simulink model "newsyscase1modctrlflowmod"  (R2014b)
settings: Solver=ode45  StartTime=0.0  StopTime=2000  RelTol=1e-3
values from neighbouring files (symbols this model uses):
  Dsteptime = 1000    [mainrun.m]
undefined symbols (not defined in the file or in its folder): D1, D10, D11, D12, D2, D3, D4, D5, D6, D7, D8, D9, Is1, Is2, Is3, Is4, Ks1, Ks2, Ks3, Ks4
undefined symbols (not defined in the file): H1C1initT, H1C2initT, H2C1initT, H2C2initT, H2C3initT, Ttank1, Ttank2, Ttank3, Ttank4, Ttank5
libraries: simulink x4, commblkintrlv2 x1
settings Model: Creator=fredrik  LastModifiedBy=fredrik

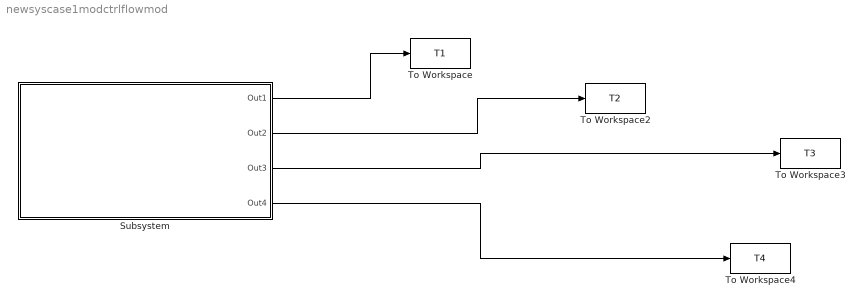
== system newsyscase1modctrlflowmod ==
  Subsystem : Subsystem
  To Workspace : ToWorkspace  VariableName=T1  SaveFormat=Timeseries  SampleTime=-1
  To Workspace2 : ToWorkspace  VariableName=T2  SaveFormat=Timeseries  SampleTime=-1
  To Workspace3 : ToWorkspace  VariableName=T3  SaveFormat=Timeseries  SampleTime=-1
  To Workspace4 : ToWorkspace  VariableName=T4  SaveFormat=Timeseries  SampleTime=-1
  wires:
  Subsystem/1(Out1) -> To Workspace/1
  Subsystem/2(Out2) -> To Workspace2/1
  Subsystem/3(Out3) -> To Workspace3/1
  Subsystem/4(Out4) -> To Workspace4/1

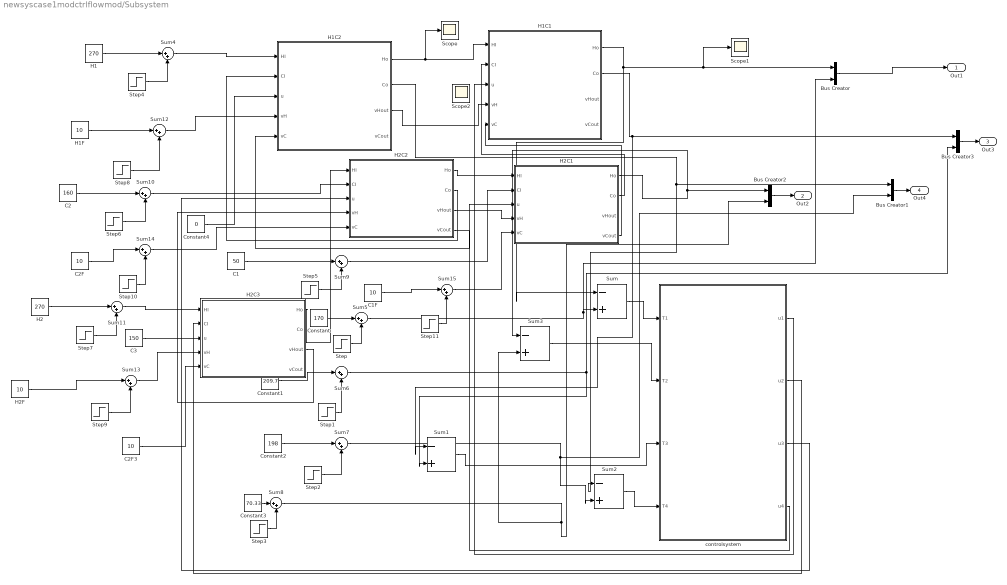
== system newsyscase1modctrlflowmod/Subsystem ==
  Bus Creator{,1..3} (4 alike) : BusCreator  Inputs=2
  C1 : Constant  Value=50
  C1F : Constant  Value=10
  C2 : Constant  Value=160
  C2F : Constant  Value=10
  C2F3 : Constant  Value=10
  C3 : Constant  Value=150
  Constant : Constant  Value=170
  Constant1 : Constant  Value=209.7
  Constant2 : Constant  Value=198
  Constant3 : Constant  Value=70.33
  Constant4 : Constant  Value=0
  H1 : Constant  Value=270
  H1C1 : Subsystem  mask{A=239.1281493, Vhot=Ttank2*10, Vcold=Ttank2*10, Q=1000, Ulm=0.5, Thin=225.55555, Thout=170, Tcin=160, Tcout=210, vh=10, vc=10, n=10, initT=H1C1initT, hot=1}
      mask prompts: A "Area"; Vhot "Volume for hot stream"; Vcold "Volume for cold stream"; Ulm "U"; Thin "Hotin"; Thout "Hotout"; Tcin "Coldin"; Tcout "Coldout"; vh "Rated hot flow"; vc "Rated cold flow"; n "Number of cells"; initT "initial temperature"; hot "1 if hot bypass, 0 if cold"
      mask init:
      | % vH=sym('vH');
      | % Vh=sym('Vh');
      | % th=sym('th');
      | % u0=sym('u0'); %
      | % Vend=sym('Vend');
      | % vC=sym('vC');
      | % Vc=sym('Vc');
      | % tc=sym('tc');
      | 
      | %%tank1:
      | 
      | %% E-2401
      | Fc=Q/(Tcout-Tcin)/vc;
      | Fh=Q/(Thin-Thout)/vh;
      | %Fsak=2*1/(1/Fc+1/Fh);
      | %Nth=Ulm*A/Fsak;
      | %U=Ulm/(n-Nth)*n;
      | %UA=A*U;
      | tc=1/(A/(Fc*Vcold));%cold constant for transfer
      | th=1/(A/(Fh*Vhot));%hot constant for transfer
      | Am=zeros(2*n+1);
      | AU=zeros(2*n+1);
      | Avhot=zeros(2*n+1);
      | Avcold=zeros(2*n+1);
      | Ath=zeros(2*n+1);
      | B=zeros(2*n,1);
      | C=zeros(2,2*n+1);
      | if hot
      |     C(2,end)=1;
      |     C(1,2)=1;
      | else
      |     C(1,end)=1;
      |     C(2,end-2)=1;
      | end
      | D=zeros(2*n,1);
      | 
      | 
      | for k=1:2*n
      |     if mod(k,2) == 1
      |         Ath(k,k)=-1/th;
      |         Am(k,k)=-n/Vhot;
      |         Avhot(k,k)=1;
      |         Ath(k,k+1)=1/th;
      |         if hot
      |             AU(k,k)=n/Vhot;
      |         end
      |         if k~=1
      |             Am(k,k-2)=n/Vhot;
      |             if hot
      |                 AU(k,k-2)=-n/Vhot;
      |             end
      |         end
      |     else
      |         Ath(k,k)=-1/tc;
      |         Avcold(k,k)=1;
      |         Am(k,k)=-n/Vcold;
      |         Ath(k,k-1)=1/tc;
      |         if ~hot
      |             AU(k,k)=n/Vcold;
      |         end
      |         if k~=2*n
      |             Am(k,k+2)=n/Vcold;
      |             if ~hot
      |                 AU(k,k+2)=-n/Vcold;
      |             end
      |         end
      |     end
      | end
      | ADscold=zeros(2*n+1);
      | ADshot=zeros(2*n+1);
      | Ds=zeros(2*n+1,2);
      | %Ds=sym(Ds);
      | Ds(1,1)=(n/Vhot);
      | ADshot(1,1)=1;
      | Ds(2*n,2)=(n/Vcold);
      | ADscold(2*n,2*n)=1;
      | DsU=zeros(2*n+1,2);
      | %DsU=sym(DsU);
      | if hot
      |     DsU(1,1)=(-n/Vhot);
      | else
      |     DsU(2*n,2)=(-n/Vcold);
      | end
      | 
      | 
      | if hot
      |     Am(2*n+1,end-2)=n/Vhot;
      |     AU(2*n+1,end-2)=-n/Vhot;
      |     Am(2*n+1,end)=-n/Vhot;
      |     Avhot(end,end)=1;
      |     DsU(end,1)=n/Vhot;
      |     ADshot(end,end)=1;
      | else
      |     Am(2*n+1,2)=n/Vcold;
      |     Am(2*n+1,end)=-n/Vcold;
      |     AU(2*n+1,2)=-n/Vcold;
      |     Avcold(end,end)=1;
      |     DsU(end,2)=n/Vcold;
      |     ADscold(end,end)=1;
      | end
      | %DsU(end,1)=1;
      | %A(2*n+1,end-2)=1;
      | %AU(2*n+1,end-2)=-1;
      | 
      | 
      | 
      | % x=zeroes(10000,2*n);
      | % k=0:0.1:1000;
      | % X=zeroes(10000,2*n);
      | % X(1,:)=initT;
      | % for k=0:1:10000;
      | %
      | % end
      | %
      | % X=A*X+Ds*TI;
      | 
      | 
      | %A=[-(3*vH/Vh*(1-u0)+1/th) 1/th 0 0 0 0 0; 1/tc -(3*vC/Vc+1/tc) 0 3*vC/Vc 0 0 0; 3*vH/Vh*(1-u0) 0 -(3*vH/Vh*(1-u0)+1/th) 1/th 0 0 0; 0 0 1/tc -(3*vC/Vc+1/tc) 0 3*vC/Vc 0;0 0 3*vH/Vh*(1-u0) 0 -(3*vH/Vh*(1-u0)+1/th) 1/th 0;0 0 0 0 1/tc -(3*vC/Vc+1/tc) 0; 0 0 0 0 (1-u0)*vH/Vend 0 -vH/Vend];A
  H1C2 : Subsystem  mask{A=28.27287318, Vhot=Ttank1*10, Vcold=Ttank1*10, Q=800, Ulm=0.5, Thin=270, Thout=225.5555, Tcin=182, Tcout=198, vh=10, vc=10, n=10, initT=H1C2initT, hot=1}
      mask prompts: A "Area"; Vhot "Volume for hot stream"; Vcold "Volume for cold stream"; Ulm "U"; Thin "Hotin"; Thout "Hotout"; Tcin "Coldin"; Tcout "Coldout"; vh "Rated hot flow"; vc "Rated cold flow"; n "Number of cells"; initT "initial temperature"; hot "1 if hot bypass, 0 if cold"
      mask init: same as newsyscase1modctrlflowmod/Subsystem/H1C1
  H1F : Constant  Value=10
  H2 : Constant  Value=270
  H2C1 : Subsystem  mask{A=466.4208212, Vhot=Ttank4*10, Vcold=Ttank4*10, Q=2200, Ulm=0.5, Thin=170, Thout=70, Tcin=50, Tcout=160, vh=10, vc=10, n=15, initT=H2C1initT, hot=1}
      mask prompts: A "Area"; Vhot "Volume for hot stream"; Vcold "Volume for cold stream"; Ulm "U"; Thin "Hotin"; Thout "Hotout"; Tcin "Coldin"; Tcout "Coldout"; vh "Rated hot flow"; vc "Rated cold flow"; n "Number of cells"; initT "initial temperature"; hot "1 if hot bypass, 0 if cold"
      mask init: same as newsyscase1modctrlflowmod/Subsystem/H1C1
  H2C2 : Subsystem  mask{A=140.693508, Vhot=Ttank3*10, Vcold=Ttank3*10, Q=1100, Ulm=0.5, Thin=220, Thout=170, Tcin=160, Tcout=182, vh=10, vc=10, n=10, initT=H2C2initT, hot=1}
      mask prompts: A "Area"; Vhot "Volume for hot stream"; Vcold "Volume for cold stream"; Ulm "U"; Thin "Hotin"; Thout "Hotout"; Tcin "Coldin"; Tcout "Coldout"; vh "Rated hot flow"; vc "Rated cold flow"; n "Number of cells"; initT "initial temperature"; hot "1 if hot bypass, 0 if cold"
      mask init: same as newsyscase1modctrlflowmod/Subsystem/H1C1
  H2C3 : Subsystem  mask{A=57.91852701, Vhot=Ttank5*10, Vcold=Ttank5*10, Q=1100, Ulm=0.5, Thin=270, Thout=220, Tcin=150, Tcout=250, vh=10, vc=10, n=10, initT=H2C3initT, hot=1}
      mask prompts: A "Area"; Vhot "Volume for hot stream"; Vcold "Volume for cold stream"; Ulm "U"; Thin "Hotin"; Thout "Hotout"; Tcin "Coldin"; Tcout "Coldout"; vh "Rated hot flow"; vc "Rated cold flow"; n "Number of cells"; initT "initial temperature"; hot "1 if hot bypass, 0 if cold"
      mask init: same as newsyscase1modctrlflowmod/Subsystem/H1C1
  H2F : Constant  Value=10
  Scope : Scope
      settings: SaveName=ScopeData10
  Scope1 : Scope
      settings: SaveName=ScopeData11
  Scope2 : Scope
      settings: SaveName=ScopeData12
  Step : Step  Time=Dsteptime  After=D1  SampleTime=0
  Step1 : Step  Time=Dsteptime  After=D2  SampleTime=0
  Step10 : Step  Time=Dsteptime  After=D11  SampleTime=0
  Step11 : Step  Time=Dsteptime  After=D12  SampleTime=0
  Step2 : Step  Time=Dsteptime  After=D3  SampleTime=0
  Step3 : Step  Time=Dsteptime  After=D4  SampleTime=0
  Step4 : Step  Time=Dsteptime  After=D5  SampleTime=0
  Step5 : Step  Time=Dsteptime  After=D6  SampleTime=0
  Step6 : Step  Time=Dsteptime  After=D7  SampleTime=0
  Step7 : Step  Time=Dsteptime  After=D8  SampleTime=0
  Step8 : Step  Time=Dsteptime  After=D9  SampleTime=0
  Step9 : Step  Time=Dsteptime  After=D10  SampleTime=0
  Sum{,1..3} (4 alike) : Sum  Inputs=|-+
  Sum{4..15} (12 alike) : Sum  Inputs=|++
  controlsystem : Subsystem
  Out1 : Outport
  Out2 : Outport  Port=2
  Out3 : Outport  Port=3
  Out4 : Outport  Port=4
  wires:
  H2C1/1(Ho) -> Bus Creator2/1, Sum3/1
  H2C1/2(Co) -> H1C1/2(CI)
  H2C2/2(Co) -> H1C2/2(CI)
  H1C1/1(Ho) -> Scope1/1, Bus Creator/1, Sum/1
  C3/1 -> H2C3/2(CI)
  H1C2/1(Ho) -> H1C1/1(HI), Scope/1
  H2C2/1(Ho) -> H2C1/1(HI)
  H2C3/1(Ho) -> H2C2/1(HI)
  H1C2/2(Co) -> Bus Creator1/1, Sum2/1
  Constant4/1 -> H1C2/3(u)
  Sum5/1 -> Bus Creator/2, Sum/2
  Sum/1 -> controlsystem/1(T1)
  Sum6/1 -> Sum1/2, Bus Creator3/2
  Sum7/1 -> Bus Creator1/2, Sum2/2
  Sum8/1 -> Bus Creator2/2, Sum3/2
  Sum1/1 -> controlsystem/3(T3)
  Sum2/1 -> controlsystem/4(T4)
  Sum3/1 -> controlsystem/2(T2)
  Bus Creator/1 -> Out1/1
  H1C1/2(Co) -> Bus Creator3/1, Sum1/1
  Bus Creator3/1 -> Out3/1
  Bus Creator1/1 -> Out4/1
  Bus Creator2/1 -> Out2/1
  Constant3/1 -> Sum8/1
  Constant2/1 -> Sum7/1
  Constant1/1 -> Sum6/1
  Constant/1 -> Sum5/1
  Step/1 -> Sum5/2
  Step1/1 -> Sum6/2
  Step2/1 -> Sum7/2
  Step3/1 -> Sum8/2
  Step4/1 -> Sum4/2
  Step5/1 -> Sum9/2
  H1/1 -> Sum4/1
  Sum4/1 -> H1C2/1(HI)
  Sum9/1 -> H2C1/2(CI)
  C1/1 -> Sum9/1
  Step6/1 -> Sum10/2
  C2/1 -> Sum10/1
  Sum10/1 -> H2C2/2(CI)
  Step7/1 -> Sum11/2
  H2/1 -> Sum11/1
  Sum11/1 -> H2C3/1(HI)
  H1C2/3(vHout) -> H1C1/4(vH)
  H2C3/3(vHout) -> H2C2/4(vH)
  H2C2/3(vHout) -> H2C1/4(vH)
  H2C1/4(vCout) -> H1C1/5(vC)
  H2C2/4(vCout) -> H1C2/5(vC)
  C2F3/1 -> H2C3/5(vC)
  H1F/1 -> Sum12/1
  Sum12/1 -> H1C2/4(vH)
  Step8/1 -> Sum12/2
  Step9/1 -> Sum13/2
  H2F/1 -> Sum13/1
  Sum13/1 -> H2C3/4(vH)
  C2F/1 -> Sum14/1
  Sum14/1 -> H2C2/5(vC)
  Step10/1 -> Sum14/2
  Step11/1 -> Sum15/2
  C1F/1 -> Sum15/1
  Sum15/1 -> H2C1/5(vC)
  controlsystem/1(u1) -> H1C1/3(u)
  controlsystem/2(u2) -> H2C3/3(u)
  controlsystem/3(u3) -> H2C2/3(u)
  controlsystem/4(u4) -> H2C1/3(u)

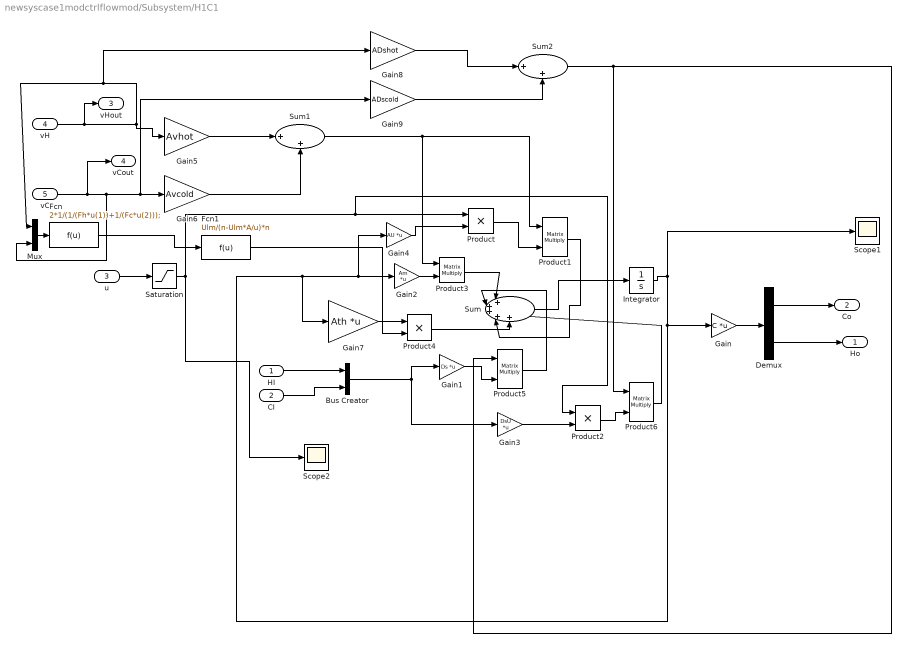
== system newsyscase1modctrlflowmod/Subsystem/H1C1 ==
  HI : Inport
  CI : Inport  Port=2
  u : Inport  Port=3
  vH : Inport  Port=4
  vC : Inport  Port=5
  Bus Creator : BusCreator  Inputs=2
  Demux : Demux  Outputs=2
  Fcn : Fcn  Expr=2*1/(1/(Fh*u(1))+1/(Fc*u(2)));
  Fcn1 : Fcn  Expr=Ulm/(n-Ulm*A/u)*n
  Gain : Gain  Gain=C  Multiplication=Matrix(K*u)
  Gain1 : Gain  Gain=Ds  Multiplication=Matrix(K*u)
  Gain2 : Gain  Gain=Am  Multiplication=Matrix(K*u)
  Gain3 : Gain  Gain=DsU  Multiplication=Matrix(K*u)
  Gain4 : Gain  Gain=AU  Multiplication=Matrix(K*u)
  Gain5 : Gain  Gain=Avhot
  Gain6 : Gain  Gain=Avcold
  Gain7 : Gain  Gain=Ath  Multiplication=Matrix(K*u)
  Gain8 : Gain  Gain=ADshot
  Gain9 : Gain  Gain=ADscold
  Integrator : Integrator  InitialCondition=initT
  Mux : Mux  Inputs=2
  Product : Product
  Product{1,3,5..6} (4 alike) : Product  Multiplication=Matrix(*)
  Product2 : Product
  Product4 : Product
  Saturation : Saturate  UpperLimit=1  LowerLimit=0
  Scope1 : Scope
      settings: ShowLegends=on  YMin=60  YMax=220  SaveName=ScopeData4
  Scope2 : Scope
      settings: SaveName=ScopeData2
  Sum : Sum  Inputs=|+++++
  Sum1 : Sum  Inputs=|++
  Sum2 : Sum  Inputs=|++
  Ho : Outport
  Co : Outport  Port=2
  vHout : Outport  Port=3
  vCout : Outport  Port=4
  wires:
  Integrator/1 -> Gain7/1, Gain4/1, Gain2/1, Gain/1, Scope1/1
  Sum/1 -> Integrator/1
  Bus Creator/1 -> Gain1/1, Gain3/1
  Gain3/1 -> Product2/2
  Gain4/1 -> Product/2
  Saturation/1 -> Product2/1, Product/1, Scope2/1
  HI/1 -> Bus Creator/1
  CI/1 -> Bus Creator/2
  Demux/2 -> Ho/1
  Demux/1 -> Co/1
  Gain/1 -> Demux/1
  u/1 -> Saturation/1
  vH/1 -> vHout/1, Gain5/1, Gain8/1, Mux/1
  vC/1 -> vCout/1, Mux/2, Gain9/1, Gain6/1
  Gain5/1 -> Sum1/1
  Gain6/1 -> Sum1/2
  Product/1 -> Product1/2
  Sum1/1 -> Product3/1, Product1/1
  Product1/1 -> Sum/4
  Gain2/1 -> Product3/2
  Product3/1 -> Sum/1
  Gain7/1 -> Product4/1
  Product4/1 -> Sum/5
  Fcn1/1 -> Product4/2
  Mux/1 -> Fcn/1
  Fcn/1 -> Fcn1/1
  Gain8/1 -> Sum2/1
  Gain9/1 -> Sum2/2
  Gain1/1 -> Product5/2
  Sum2/1 -> Product6/1, Product5/1
  Product5/1 -> Sum/2
  Product2/1 -> Product6/2
  Product6/1 -> Sum/3

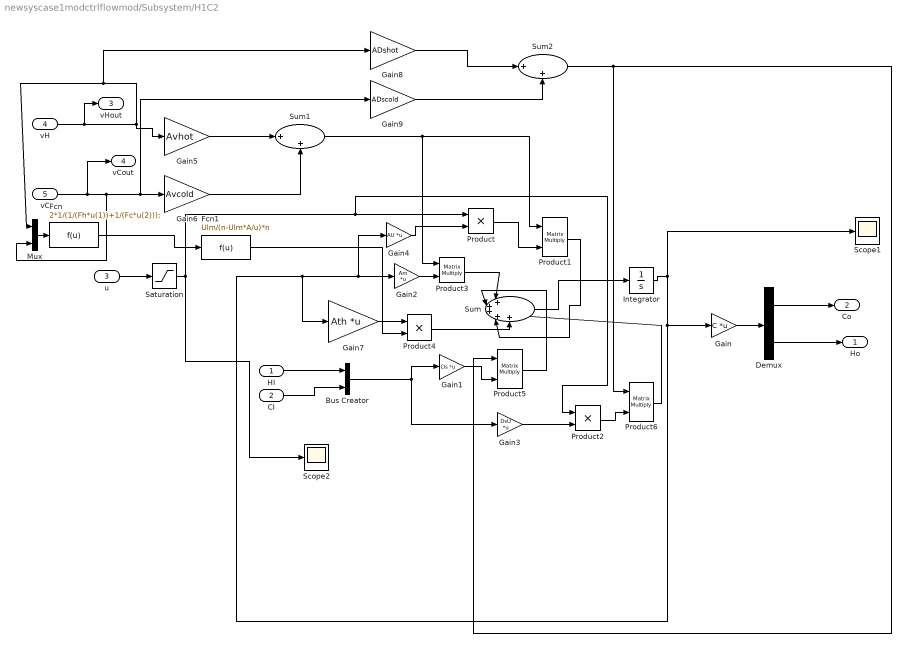
== system newsyscase1modctrlflowmod/Subsystem/H1C2 ==
  HI : Inport
  CI : Inport  Port=2
  u : Inport  Port=3
  vH : Inport  Port=4
  vC : Inport  Port=5
  Bus Creator : BusCreator  Inputs=2
  Demux : Demux  Outputs=2
  Fcn : Fcn  Expr=2*1/(1/(Fh*u(1))+1/(Fc*u(2)));
  Fcn1 : Fcn  Expr=Ulm/(n-Ulm*A/u)*n
  Gain : Gain  Gain=C  Multiplication=Matrix(K*u)
  Gain1 : Gain  Gain=Ds  Multiplication=Matrix(K*u)
  Gain2 : Gain  Gain=Am  Multiplication=Matrix(K*u)
  Gain3 : Gain  Gain=DsU  Multiplication=Matrix(K*u)
  Gain4 : Gain  Gain=AU  Multiplication=Matrix(K*u)
  Gain5 : Gain  Gain=Avhot
  Gain6 : Gain  Gain=Avcold
  Gain7 : Gain  Gain=Ath  Multiplication=Matrix(K*u)
  Gain8 : Gain  Gain=ADshot
  Gain9 : Gain  Gain=ADscold
  Integrator : Integrator  InitialCondition=initT
  Mux : Mux  Inputs=2
  Product : Product
  Product{1,3,5..6} (4 alike) : Product  Multiplication=Matrix(*)
  Product2 : Product
  Product4 : Product
  Saturation : Saturate  UpperLimit=1  LowerLimit=0
  Scope1 : Scope
      settings: ShowLegends=on  YMin=60  YMax=220  SaveName=ScopeData4
  Scope2 : Scope
      settings: SaveName=ScopeData2
  Sum : Sum  Inputs=|+++++
  Sum1 : Sum  Inputs=|++
  Sum2 : Sum  Inputs=|++
  Ho : Outport
  Co : Outport  Port=2
  vHout : Outport  Port=3
  vCout : Outport  Port=4
  wires:
  Integrator/1 -> Gain7/1, Gain4/1, Gain2/1, Gain/1, Scope1/1
  Sum/1 -> Integrator/1
  Bus Creator/1 -> Gain1/1, Gain3/1
  Gain3/1 -> Product2/2
  Gain4/1 -> Product/2
  Saturation/1 -> Product2/1, Product/1, Scope2/1
  HI/1 -> Bus Creator/1
  CI/1 -> Bus Creator/2
  Demux/2 -> Ho/1
  Demux/1 -> Co/1
  Gain/1 -> Demux/1
  u/1 -> Saturation/1
  vH/1 -> vHout/1, Gain5/1, Gain8/1, Mux/1
  vC/1 -> vCout/1, Mux/2, Gain9/1, Gain6/1
  Gain5/1 -> Sum1/1
  Gain6/1 -> Sum1/2
  Product/1 -> Product1/2
  Sum1/1 -> Product3/1, Product1/1
  Product1/1 -> Sum/4
  Gain2/1 -> Product3/2
  Product3/1 -> Sum/1
  Gain7/1 -> Product4/1
  Product4/1 -> Sum/5
  Fcn1/1 -> Product4/2
  Mux/1 -> Fcn/1
  Fcn/1 -> Fcn1/1
  Gain8/1 -> Sum2/1
  Gain9/1 -> Sum2/2
  Gain1/1 -> Product5/2
  Sum2/1 -> Product6/1, Product5/1
  Product5/1 -> Sum/2
  Product2/1 -> Product6/2
  Product6/1 -> Sum/3

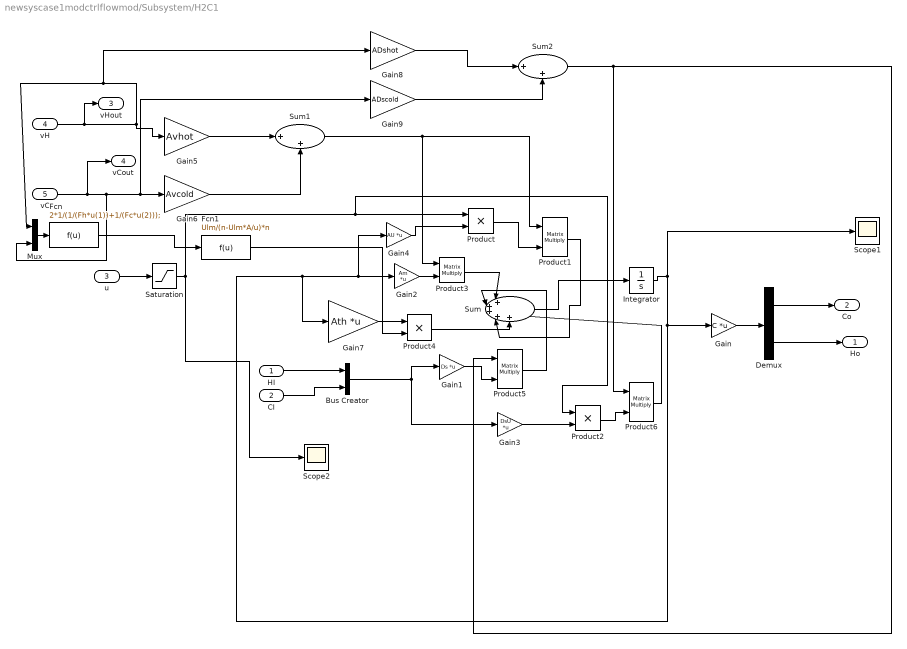
== system newsyscase1modctrlflowmod/Subsystem/H2C1 ==
  HI : Inport
  CI : Inport  Port=2
  u : Inport  Port=3
  vH : Inport  Port=4
  vC : Inport  Port=5
  Bus Creator : BusCreator  Inputs=2
  Demux : Demux  Outputs=2
  Fcn : Fcn  Expr=2*1/(1/(Fh*u(1))+1/(Fc*u(2)));
  Fcn1 : Fcn  Expr=Ulm/(n-Ulm*A/u)*n
  Gain : Gain  Gain=C  Multiplication=Matrix(K*u)
  Gain1 : Gain  Gain=Ds  Multiplication=Matrix(K*u)
  Gain2 : Gain  Gain=Am  Multiplication=Matrix(K*u)
  Gain3 : Gain  Gain=DsU  Multiplication=Matrix(K*u)
  Gain4 : Gain  Gain=AU  Multiplication=Matrix(K*u)
  Gain5 : Gain  Gain=Avhot
  Gain6 : Gain  Gain=Avcold
  Gain7 : Gain  Gain=Ath  Multiplication=Matrix(K*u)
  Gain8 : Gain  Gain=ADshot
  Gain9 : Gain  Gain=ADscold
  Integrator : Integrator  InitialCondition=initT
  Mux : Mux  Inputs=2
  Product : Product
  Product{1,3,5..6} (4 alike) : Product  Multiplication=Matrix(*)
  Product2 : Product
  Product4 : Product
  Saturation : Saturate  UpperLimit=1  LowerLimit=0
  Scope1 : Scope
      settings: ShowLegends=on  YMin=60  YMax=220  SaveName=ScopeData4
  Scope2 : Scope
      settings: SaveName=ScopeData2
  Sum : Sum  Inputs=|+++++
  Sum1 : Sum  Inputs=|++
  Sum2 : Sum  Inputs=|++
  Ho : Outport
  Co : Outport  Port=2
  vHout : Outport  Port=3
  vCout : Outport  Port=4
  wires:
  Integrator/1 -> Gain7/1, Gain4/1, Gain2/1, Gain/1, Scope1/1
  Sum/1 -> Integrator/1
  Bus Creator/1 -> Gain1/1, Gain3/1
  Gain3/1 -> Product2/2
  Gain4/1 -> Product/2
  Saturation/1 -> Product2/1, Product/1, Scope2/1
  HI/1 -> Bus Creator/1
  CI/1 -> Bus Creator/2
  Demux/2 -> Ho/1
  Demux/1 -> Co/1
  Gain/1 -> Demux/1
  u/1 -> Saturation/1
  vH/1 -> vHout/1, Gain5/1, Gain8/1, Mux/1
  vC/1 -> vCout/1, Mux/2, Gain9/1, Gain6/1
  Gain5/1 -> Sum1/1
  Gain6/1 -> Sum1/2
  Product/1 -> Product1/2
  Sum1/1 -> Product3/1, Product1/1
  Product1/1 -> Sum/4
  Gain2/1 -> Product3/2
  Product3/1 -> Sum/1
  Gain7/1 -> Product4/1
  Product4/1 -> Sum/5
  Fcn1/1 -> Product4/2
  Mux/1 -> Fcn/1
  Fcn/1 -> Fcn1/1
  Gain8/1 -> Sum2/1
  Gain9/1 -> Sum2/2
  Gain1/1 -> Product5/2
  Sum2/1 -> Product6/1, Product5/1
  Product5/1 -> Sum/2
  Product2/1 -> Product6/2
  Product6/1 -> Sum/3

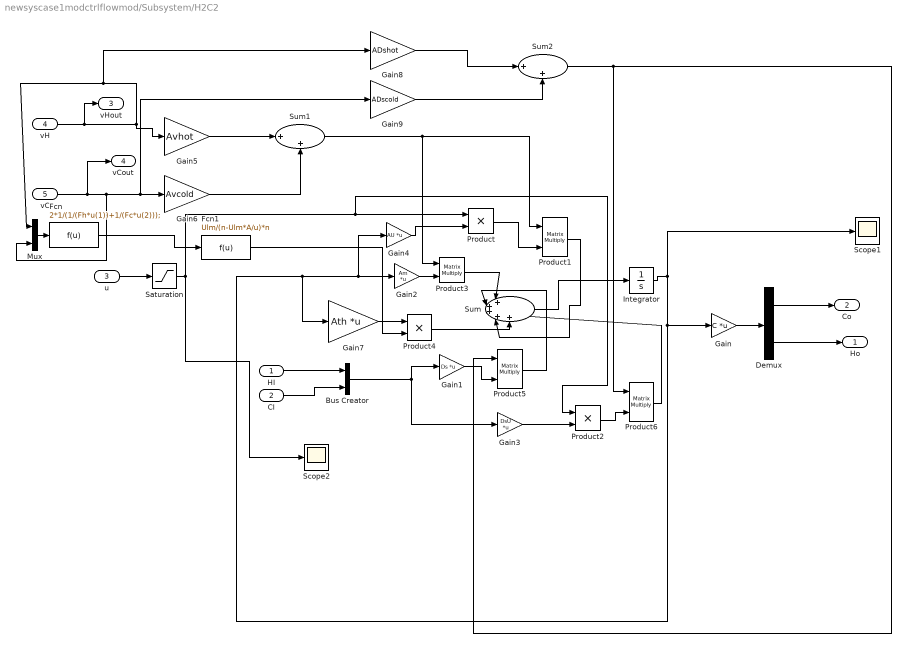
== system newsyscase1modctrlflowmod/Subsystem/H2C2 ==
  HI : Inport
  CI : Inport  Port=2
  u : Inport  Port=3
  vH : Inport  Port=4
  vC : Inport  Port=5
  Bus Creator : BusCreator  Inputs=2
  Demux : Demux  Outputs=2
  Fcn : Fcn  Expr=2*1/(1/(Fh*u(1))+1/(Fc*u(2)));
  Fcn1 : Fcn  Expr=Ulm/(n-Ulm*A/u)*n
  Gain : Gain  Gain=C  Multiplication=Matrix(K*u)
  Gain1 : Gain  Gain=Ds  Multiplication=Matrix(K*u)
  Gain2 : Gain  Gain=Am  Multiplication=Matrix(K*u)
  Gain3 : Gain  Gain=DsU  Multiplication=Matrix(K*u)
  Gain4 : Gain  Gain=AU  Multiplication=Matrix(K*u)
  Gain5 : Gain  Gain=Avhot
  Gain6 : Gain  Gain=Avcold
  Gain7 : Gain  Gain=Ath  Multiplication=Matrix(K*u)
  Gain8 : Gain  Gain=ADshot
  Gain9 : Gain  Gain=ADscold
  Integrator : Integrator  InitialCondition=initT
  Mux : Mux  Inputs=2
  Product : Product
  Product{1,3,5..6} (4 alike) : Product  Multiplication=Matrix(*)
  Product2 : Product
  Product4 : Product
  Saturation : Saturate  UpperLimit=1  LowerLimit=0
  Scope1 : Scope
      settings: ShowLegends=on  YMin=60  YMax=220  SaveName=ScopeData4
  Scope2 : Scope
      settings: SaveName=ScopeData2
  Sum : Sum  Inputs=|+++++
  Sum1 : Sum  Inputs=|++
  Sum2 : Sum  Inputs=|++
  Ho : Outport
  Co : Outport  Port=2
  vHout : Outport  Port=3
  vCout : Outport  Port=4
  wires:
  Integrator/1 -> Gain7/1, Gain4/1, Gain2/1, Gain/1, Scope1/1
  Sum/1 -> Integrator/1
  Bus Creator/1 -> Gain1/1, Gain3/1
  Gain3/1 -> Product2/2
  Gain4/1 -> Product/2
  Saturation/1 -> Product2/1, Product/1, Scope2/1
  HI/1 -> Bus Creator/1
  CI/1 -> Bus Creator/2
  Demux/2 -> Ho/1
  Demux/1 -> Co/1
  Gain/1 -> Demux/1
  u/1 -> Saturation/1
  vH/1 -> vHout/1, Gain5/1, Gain8/1, Mux/1
  vC/1 -> vCout/1, Mux/2, Gain9/1, Gain6/1
  Gain5/1 -> Sum1/1
  Gain6/1 -> Sum1/2
  Product/1 -> Product1/2
  Sum1/1 -> Product3/1, Product1/1
  Product1/1 -> Sum/4
  Gain2/1 -> Product3/2
  Product3/1 -> Sum/1
  Gain7/1 -> Product4/1
  Product4/1 -> Sum/5
  Fcn1/1 -> Product4/2
  Mux/1 -> Fcn/1
  Fcn/1 -> Fcn1/1
  Gain8/1 -> Sum2/1
  Gain9/1 -> Sum2/2
  Gain1/1 -> Product5/2
  Sum2/1 -> Product6/1, Product5/1
  Product5/1 -> Sum/2
  Product2/1 -> Product6/2
  Product6/1 -> Sum/3

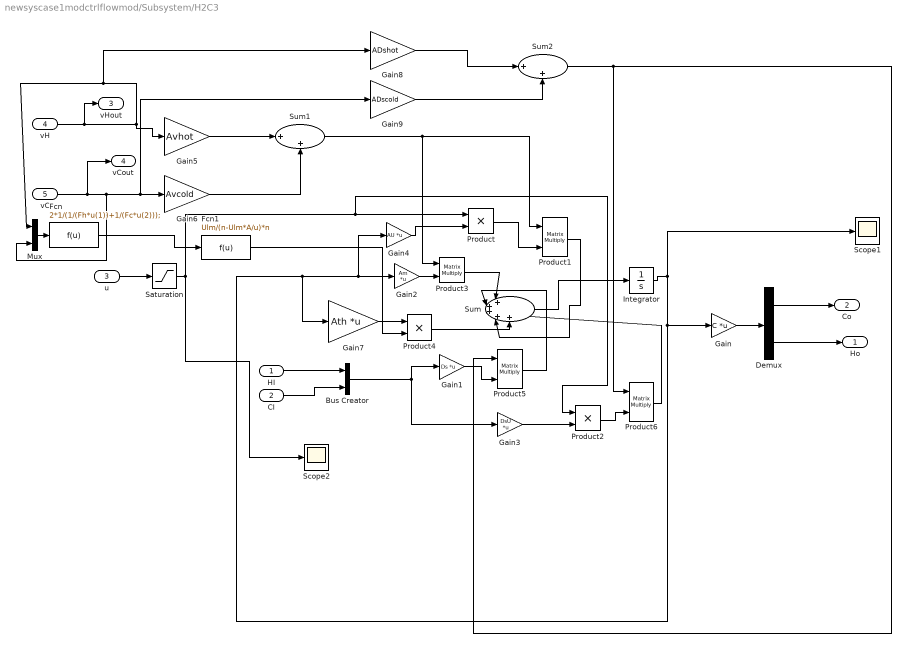
== system newsyscase1modctrlflowmod/Subsystem/H2C3 ==
  HI : Inport
  CI : Inport  Port=2
  u : Inport  Port=3
  vH : Inport  Port=4
  vC : Inport  Port=5
  Bus Creator : BusCreator  Inputs=2
  Demux : Demux  Outputs=2
  Fcn : Fcn  Expr=2*1/(1/(Fh*u(1))+1/(Fc*u(2)));
  Fcn1 : Fcn  Expr=Ulm/(n-Ulm*A/u)*n
  Gain : Gain  Gain=C  Multiplication=Matrix(K*u)
  Gain1 : Gain  Gain=Ds  Multiplication=Matrix(K*u)
  Gain2 : Gain  Gain=Am  Multiplication=Matrix(K*u)
  Gain3 : Gain  Gain=DsU  Multiplication=Matrix(K*u)
  Gain4 : Gain  Gain=AU  Multiplication=Matrix(K*u)
  Gain5 : Gain  Gain=Avhot
  Gain6 : Gain  Gain=Avcold
  Gain7 : Gain  Gain=Ath  Multiplication=Matrix(K*u)
  Gain8 : Gain  Gain=ADshot
  Gain9 : Gain  Gain=ADscold
  Integrator : Integrator  InitialCondition=initT
  Mux : Mux  Inputs=2
  Product : Product
  Product{1,3,5..6} (4 alike) : Product  Multiplication=Matrix(*)
  Product2 : Product
  Product4 : Product
  Saturation : Saturate  UpperLimit=1  LowerLimit=0
  Scope1 : Scope
      settings: ShowLegends=on  YMin=60  YMax=220  SaveName=ScopeData4
  Scope2 : Scope
      settings: SaveName=ScopeData2
  Sum : Sum  Inputs=|+++++
  Sum1 : Sum  Inputs=|++
  Sum2 : Sum  Inputs=|++
  Ho : Outport
  Co : Outport  Port=2
  vHout : Outport  Port=3
  vCout : Outport  Port=4
  wires:
  Integrator/1 -> Gain7/1, Gain4/1, Gain2/1, Gain/1, Scope1/1
  Sum/1 -> Integrator/1
  Bus Creator/1 -> Gain1/1, Gain3/1
  Gain3/1 -> Product2/2
  Gain4/1 -> Product/2
  Saturation/1 -> Product2/1, Product/1, Scope2/1
  HI/1 -> Bus Creator/1
  CI/1 -> Bus Creator/2
  Demux/2 -> Ho/1
  Demux/1 -> Co/1
  Gain/1 -> Demux/1
  u/1 -> Saturation/1
  vH/1 -> vHout/1, Gain5/1, Gain8/1, Mux/1
  vC/1 -> vCout/1, Mux/2, Gain9/1, Gain6/1
  Gain5/1 -> Sum1/1
  Gain6/1 -> Sum1/2
  Product/1 -> Product1/2
  Sum1/1 -> Product3/1, Product1/1
  Product1/1 -> Sum/4
  Gain2/1 -> Product3/2
  Product3/1 -> Sum/1
  Gain7/1 -> Product4/1
  Product4/1 -> Sum/5
  Fcn1/1 -> Product4/2
  Mux/1 -> Fcn/1
  Fcn/1 -> Fcn1/1
  Gain8/1 -> Sum2/1
  Gain9/1 -> Sum2/2
  Gain1/1 -> Product5/2
  Sum2/1 -> Product6/1, Product5/1
  Product5/1 -> Sum/2
  Product2/1 -> Product6/2
  Product6/1 -> Sum/3

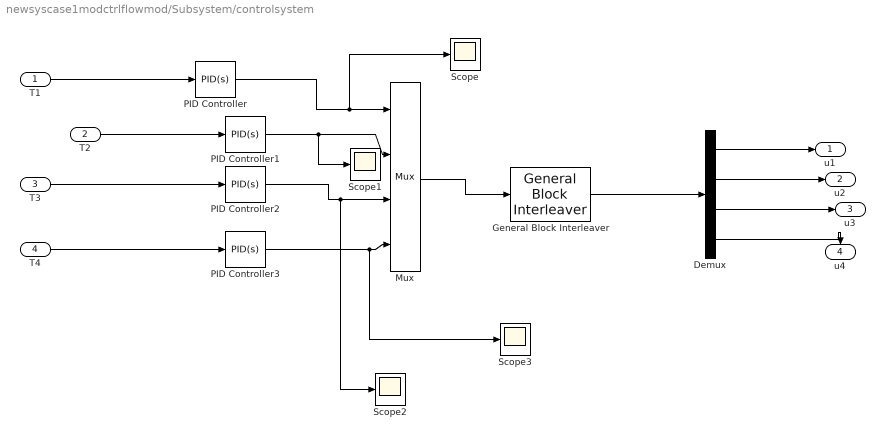
== system newsyscase1modctrlflowmod/Subsystem/controlsystem ==
  T1 : Inport
  T2 : Inport  Port=2
  T3 : Inport  Port=3
  T4 : Inport  Port=4
  Demux : Demux
  General Block Interleaver : commblkintrlv2/General Block Interleaver  permutationVectorSource=Dialog  elements=IndexG
  Mux : Mux
  PID Controller : simulink/Continuous/PID Controller  Controller=PID  TimeDomain=Continuous-time  SampleTime=-1  IntegratorMethod=Forward Euler  FilterMethod=Forward Euler  Form=Parallel  P=Ks1  I=Is1  D=0  N=100  InitialConditionSource=internal  InitialConditionForIntegrator=0.1  InitialConditionForFilter=0  ExternalReset=none  LimitOutput=on  UpperSaturationLimit=1  LowerSaturationLimit=0  LinearizeAsGain=on  AntiWindupMode=clamping  Kb=1  TrackingMode=off  Kt=1  PParamMin=[]  PParamMax=[]  IParamMin=[]  IParamMax=[]  DParamMin=[]  DParamMax=[]  NParamMin=[]  NParamMax=[]  KbParamMin=[]  KbParamMax=[]  KtParamMin=[]  KtParamMax=[]  POutMin=[]  POutMax=[]  IOutMin=[]  IOutMax=[]  DOutMin=[]  DOutMax=[]  NOutMin=[]  NOutMax=[]  KbOutMin=[]  KbOutMax=[]  KtOutMin=[]  KtOutMax=[]  IntegratorOutMin=[]  IntegratorOutMax=[]  FilterOutMin=[]  FilterOutMax=[]  SumOutMin=[]  SumOutMax=[]  SumI1OutMin=[]  SumI1OutMax=[]  SumI2OutMin=[]  SumI2OutMax=[]  SumI3OutMin=[]  SumI3OutMax=[]  SumDOutMin=[]  SumDOutMax=[]  SaturationOutMin=[]  SaturationOutMax=[]  IntegratorContinuousStateAttributes=''  IntegratorStateMustResolveToSignalObject=off  IntegratorRTWStateStorageClass=Auto  FilterContinuousStateAttributes=''  FilterStateMustResolveToSignalObject=off  FilterRTWStateStorageClass=Auto  DifferentiatorICPrevScaledInput=0  DifferentiatorOutMin=[]  DifferentiatorOutMax=[]  UseFilter=on
  PID Controller1 : simulink/Continuous/PID Controller  Controller=PID  TimeDomain=Continuous-time  SampleTime=-1  IntegratorMethod=Forward Euler  FilterMethod=Forward Euler  Form=Parallel  P=Ks2  I=Is2  D=0  N=100  InitialConditionSource=internal  InitialConditionForIntegrator=0.1  InitialConditionForFilter=0  ExternalReset=none  LimitOutput=on  UpperSaturationLimit=1  LowerSaturationLimit=0  LinearizeAsGain=on  AntiWindupMode=clamping  Kb=1  TrackingMode=off  Kt=1  PParamMin=[]  PParamMax=[]  IParamMin=[]  IParamMax=[]  DParamMin=[]  DParamMax=[]  NParamMin=[]  NParamMax=[]  KbParamMin=[]  KbParamMax=[]  KtParamMin=[]  KtParamMax=[]  POutMin=[]  POutMax=[]  IOutMin=[]  IOutMax=[]  DOutMin=[]  DOutMax=[]  NOutMin=[]  NOutMax=[]  KbOutMin=[]  KbOutMax=[]  KtOutMin=[]  KtOutMax=[]  IntegratorOutMin=[]  IntegratorOutMax=[]  FilterOutMin=[]  FilterOutMax=[]  SumOutMin=[]  SumOutMax=[]  SumI1OutMin=[]  SumI1OutMax=[]  SumI2OutMin=[]  SumI2OutMax=[]  SumI3OutMin=[]  SumI3OutMax=[]  SumDOutMin=[]  SumDOutMax=[]  SaturationOutMin=[]  SaturationOutMax=[]  IntegratorContinuousStateAttributes=''  IntegratorStateMustResolveToSignalObject=off  IntegratorRTWStateStorageClass=Auto  FilterContinuousStateAttributes=''  FilterStateMustResolveToSignalObject=off  FilterRTWStateStorageClass=Auto  DifferentiatorICPrevScaledInput=0  DifferentiatorOutMin=[]  DifferentiatorOutMax=[]  UseFilter=on
  PID Controller2 : simulink/Continuous/PID Controller  Controller=PID  TimeDomain=Continuous-time  SampleTime=-1  IntegratorMethod=Forward Euler  FilterMethod=Forward Euler  Form=Parallel  P=Ks3  I=Is3  D=0  N=100  InitialConditionSource=internal  InitialConditionForIntegrator=0.1  InitialConditionForFilter=0  ExternalReset=none  LimitOutput=on  UpperSaturationLimit=1  LowerSaturationLimit=0  LinearizeAsGain=on  AntiWindupMode=clamping  Kb=1  TrackingMode=off  Kt=1  PParamMin=[]  PParamMax=[]  IParamMin=[]  IParamMax=[]  DParamMin=[]  DParamMax=[]  NParamMin=[]  NParamMax=[]  KbParamMin=[]  KbParamMax=[]  KtParamMin=[]  KtParamMax=[]  POutMin=[]  POutMax=[]  IOutMin=[]  IOutMax=[]  DOutMin=[]  DOutMax=[]  NOutMin=[]  NOutMax=[]  KbOutMin=[]  KbOutMax=[]  KtOutMin=[]  KtOutMax=[]  IntegratorOutMin=[]  IntegratorOutMax=[]  FilterOutMin=[]  FilterOutMax=[]  SumOutMin=[]  SumOutMax=[]  SumI1OutMin=[]  SumI1OutMax=[]  SumI2OutMin=[]  SumI2OutMax=[]  SumI3OutMin=[]  SumI3OutMax=[]  SumDOutMin=[]  SumDOutMax=[]  SaturationOutMin=[]  SaturationOutMax=[]  IntegratorContinuousStateAttributes=''  IntegratorStateMustResolveToSignalObject=off  IntegratorRTWStateStorageClass=Auto  FilterContinuousStateAttributes=''  FilterStateMustResolveToSignalObject=off  FilterRTWStateStorageClass=Auto  DifferentiatorICPrevScaledInput=0  DifferentiatorOutMin=[]  DifferentiatorOutMax=[]  UseFilter=on
  PID Controller3 : simulink/Continuous/PID Controller  Controller=PID  TimeDomain=Continuous-time  SampleTime=-1  IntegratorMethod=Forward Euler  FilterMethod=Forward Euler  Form=Parallel  P=Ks4  I=Is4  D=0  N=100  InitialConditionSource=internal  InitialConditionForIntegrator=0.1  InitialConditionForFilter=0  ExternalReset=none  LimitOutput=on  UpperSaturationLimit=1  LowerSaturationLimit=0  LinearizeAsGain=on  AntiWindupMode=clamping  Kb=1  TrackingMode=off  Kt=1  PParamMin=[]  PParamMax=[]  IParamMin=[]  IParamMax=[]  DParamMin=[]  DParamMax=[]  NParamMin=[]  NParamMax=[]  KbParamMin=[]  KbParamMax=[]  KtParamMin=[]  KtParamMax=[]  POutMin=[]  POutMax=[]  IOutMin=[]  IOutMax=[]  DOutMin=[]  DOutMax=[]  NOutMin=[]  NOutMax=[]  KbOutMin=[]  KbOutMax=[]  KtOutMin=[]  KtOutMax=[]  IntegratorOutMin=[]  IntegratorOutMax=[]  FilterOutMin=[]  FilterOutMax=[]  SumOutMin=[]  SumOutMax=[]  SumI1OutMin=[]  SumI1OutMax=[]  SumI2OutMin=[]  SumI2OutMax=[]  SumI3OutMin=[]  SumI3OutMax=[]  SumDOutMin=[]  SumDOutMax=[]  SaturationOutMin=[]  SaturationOutMax=[]  IntegratorContinuousStateAttributes=''  IntegratorStateMustResolveToSignalObject=off  IntegratorRTWStateStorageClass=Auto  FilterContinuousStateAttributes=''  FilterStateMustResolveToSignalObject=off  FilterRTWStateStorageClass=Auto  DifferentiatorICPrevScaledInput=0  DifferentiatorOutMin=[]  DifferentiatorOutMax=[]  UseFilter=on
  Scope{,1..3} (4 alike) : Scope
      Scope settings: SaveName=ScopeData6
      Scope1 settings: SaveName=ScopeData7
      Scope2 settings: SaveName=ScopeData8
      Scope3 settings: SaveName=ScopeData9
  u1 : Outport
  u2 : Outport  Port=2
  u3 : Outport  Port=3
  u4 : Outport  Port=4
  wires:
  Demux/2 -> u2/1
  Demux/1 -> u1/1
  Demux/3 -> u3/1
  Demux/4 -> u4/1
  Mux/1 -> General Block Interleaver/1
  T1/1 -> PID Controller/1
  General Block Interleaver/1 -> Demux/1
  PID Controller3/1 -> Scope3/1, Mux/4
  PID Controller/1 -> Scope/1, Mux/1
  PID Controller1/1 -> Scope1/1, Mux/2
  PID Controller2/1 -> Scope2/1, Mux/3
  T2/1 -> PID Controller1/1
  T4/1 -> PID Controller3/1
  T3/1 -> PID Controller2/1
